simulink model "SF032A_MotTqCmdSca"  (R2013b)
settings: Solver=FixedStepDiscrete  SolverMode=SingleTasking  StartTime=0.0  StopTime=10  FixedStep=0.002  RelTol=1e-3
values from neighbouring files (symbols this model uses):
  MotTqCmdScaMax = DataDict.Calibration    [SF032A_MotTqCmdSca_DataDict.m]
  MotTqCmdScaMin = DataDict.Calibration    [SF032A_MotTqCmdSca_DataDict.m]
undefined symbols (not defined in the file or in its folder): NvmGetErrSts1
libraries: simulink x6, NxtrNvM x3, NxtrLim x2
Description:
  | The EOL Torque Command Scale function multiplies the MRFMtrTrqCmd input signal by a calibration which is set during a manufacturing
  | end of line calibration process. The calibration is provided to reduce overall system output torque variation. This scaled version of the motor
  | torque command is used by SF99B - Motor Control.
settings Model: Creator=LZDRZ1  LastModifiedBy=TZ5743
settings SolverCC: AutoInsertRateTranBlk=on  InsertRTBMode=Always
settings DataIOCC: LimitDataPoints=off  SaveFormat=Structure  ReturnWorkspaceOutputs=on
settings OptimizationCC: BlockReduction=off  InlineParams=on  ZeroExternalMemoryAtStartup=off  ZeroInternalMemoryAtStartup=off  OptimizeModelRefInitCode=on  LifeSpan=1
settings DebuggingCC: SignalInfNanChecking=error  SignalRangeChecking=warning  UnderspecifiedInitializationDetection=Simplified  SolverPrmCheckMsg=error  InheritedTsInSrcMsg=error  DiscreteInheritContinuousMsg=error  SingleTaskRateTransMsg=error  TasksWithSamePriorityMsg=error  SigSpecEnsureSampleTimeMsg=error  CheckMatrixSingularityMsg=error  ParameterUnderflowMsg=error  ParameterPrecisionLossMsg=error  ParameterTunabilityLossMsg=error  FixptConstUnderflowMsg=warning  FixptConstOverflowMsg=warning  VectorMatrixConversionMsg=error  SignalLabelMismatchMsg=error  UnconnectedInputMsg=error  UnconnectedOutputMsg=error  UnconnectedLineMsg=error  SFcnCompatibilityMsg=error  UniqueDataStoreMsg=warning  BusObjectLabelMismatch=error  RootOutportRequireBusObject=error  AssertControl=DisableAll  ModelReferenceIOMsg=error  ModelReferenceVersionMismatchMessage=warning  ModelReferenceIOMismatchMessage=error  ModelReferenceCSMismatchMessage=warning  ModelReferenceDataLoggingMessage=error  StateNameClashWarn=warning  StrictBusMsg=ErrorOnBusTreatedAsVector  NonBusSignalsTreatedAsBus=error  SFUnexpectedBacktrackingDiag=error  SFInvalidInputDataAccessInChartInitDiag=error  SFNoUnconditionalDefaultTransitionDiag=error  SFTransitionOutsideNaturalParentDiag=error  SFUnconditionalTransitionShadowingDiag=error  SFUndirectedBroadcastEventsDiag=error
settings ModelReferenceCC: ModelReferenceNumInstancesAllowed=Single
settings RTWCC: SystemTargetFile=autosar.tlc  GenCodeOnly=on  TemplateMakefile=ert_default_tmf  Description=AUTOSAR  GenerateReport=on  ProcessScript=autosar_make_rtw_hook  LaunchReport=on
settings CodeAppCC: GenerateComments=off  IgnoreCustomStorageClasses=off  CustomSymbolStrType=$N$R$M  CustomSymbolStrBlkIO=$N$M  SimulinkBlockComments=off
settings STFCustomTargetCC: ParMdlRefBuildCompliant=on  CompOptLevelCompliant=on  IncludeMdlTerminateFcn=off  CombineOutputUpdateFcns=on  SuppressErrorStatus=on  ERTFirstTimeCompliant=on  ERTCustomFileBanners=on  SupportNonFinite=off  SupportComplex=off  SupportContinuousTime=off  SupportNonInlinedSFcns=off  MATLABClassNameForMDSCustomization=Simulink.SoftwareTarget.ERTCustomization  AutosarCompliant=on  GRTInterface=off  SystemTargetFile=autosar.tlc
settings ERTTargetCC: CodeReplacementLibrary=ANSI_C  ConcurrentExecutionCompliant=off  IncludeMdlTerminateFcn=off  SuppressErrorStatus=on  SupportNonFinite=off  SupportComplex=off  ModelStepFunctionPrototypeControlCompliant=off  CPPClassGenCompliant=off  AutosarCompliant=on  InlinedParameterPlacement=NonHierarchical  ERTCustomFileTemplate=example_file_process.tlc  EnableUserReplacementTypes=on

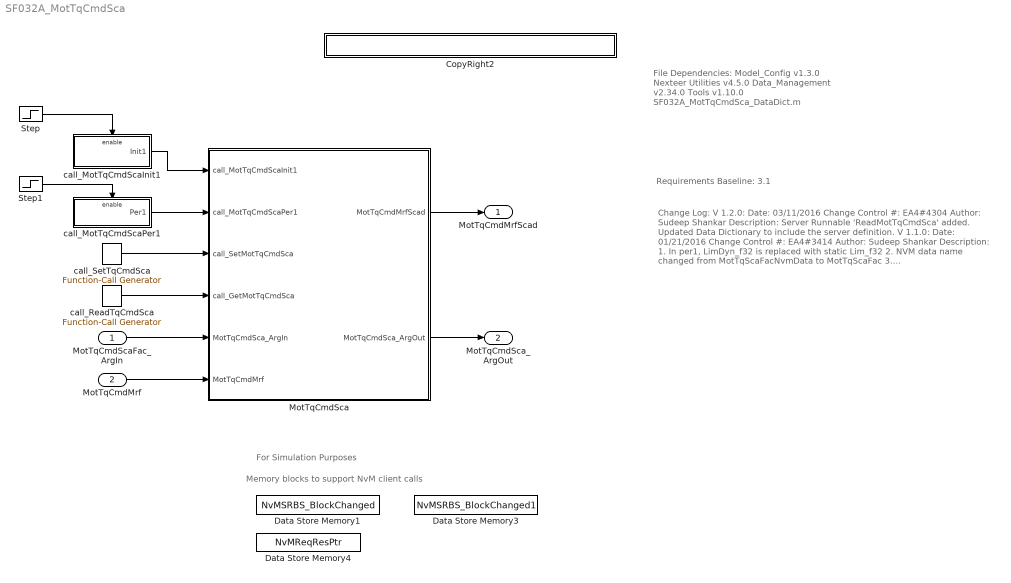
== system SF032A_MotTqCmdSca ==
  note: Change Log:
      |
      | V 1.2.0:
      | Date: 03/11/2016
      | Change Control #: EA4#4304
      | Author: Sudeep Shankar
      | Description: Server Runnable 'ReadMotTqCmdSca' added. Updated
      | Data Dictionary to include the server definition.
      |
      | V 1.1.0:
      | Date: 01/21/2016
      | Change Control #: EA4#3414
      | Author: Sudeep Shankar
      | Description:
      | 1. In per1, LimDyn_f32  is replaced with static Lim_f32
      | 2. NVM data name changed from MotTqScaFacNvmData
      |     to MotTqScaFac
      | 3. MotTqScaFacNvmData.EngInit changed from 1 to [] and ASIL
      |     level changed from 'QM' to 'D' in Data Dictionary
      | 4. SetMotTqCmdSca SrvRunnable MotTqCmdSca argument
      |     range changed in DD : EngMax = 1.1 and EngMin = 0.9
      | 5. SYSGLBPRMMOTTQCMDHILIM_MOTNWTMTR_F32
      | changed to SYSGLBPRM_MOTTQCMDHILIM_MOTNWTMTR_F32
      | 6. SYSGLBPRMMOTTQCMDLOWRLIM_MOTNWTMTR_F32
      | changed to SYSGLBPRM_MOTTQCMDLOLIM_MOTNWTMTR_F32
      |
      |
      | V 1.0.0
      | Date: 01/07/2016
      | Change Control #: EA4#2728
      | Author: Sudeep Shankar
      | Description:
      | - Initial Release Based on EA3 V 1.0.0
  note: File Dependencies:
      |
      | Model_Config v1.3.0
      | Nexteer Utilities v4.5.0
      | Data_Management v2.34.0
      | Tools v1.10.0
      | SF032A_MotTqCmdSca_DataDict.m
  note: Requirements Baseline: 3.1
  note: For Simulation Purposes
  note: Memory blocks to support NvM client calls
  MotTqCmdScaFac_ArgIn : Inport
  MotTqCmdMrf : Inport  RequirementInfo={} %GIDa_844b656b_352f_4279_ab07_8ab5443a19da  Port=2
  CopyRight2 : Subsystem  Description=|  mask(Copyright Information){none=on}
      | Copyright info block.                                               
      |                                                                     
      | Place copyright information at the top of every subsystem in design.
      mask prompts: none "No parameters"
      mask help: Place copyright information at the top of every subsystem in design.
      mask Display:
      | NxtrConf = 'Nexteer Confidential';
      | 
      | sys = bdroot; %handle for the current model ("system")
      | first = get_param(sys,'Created');
      | if(isempty(first))
      |     first = datestr(now,'yyyy');
      | else
      |     first = first(end-3:end);  %year is last four digits
      | end
      | 
      | last = get_param(sys,'LastModifiedDate');
      | if isempty(last)
      |     last = datestr(now,'yyyy');
      | else
      |     last = last(end-3:end);
      | end
      | 
      | if strcmp(first,last)
      |     fprintf('%s -- Copyright %s Nexteer',NxtrConf,first)
      | else
      |     fprintf('%s -- %s%s- %s Nexteer',NxtrConf,char(169),first,last)
      | end
  Data Store Memory1 : DataStoreMemory  DataStoreName=NvMSRBS_BlockChanged  ReadBeforeWriteMsg=warning  WriteAfterWriteMsg=warning  WriteAfterReadMsg=warning
  Data Store Memory3 : DataStoreMemory  DataStoreName=NvMSRBS_BlockChanged1  ReadBeforeWriteMsg=warning  WriteAfterWriteMsg=warning  WriteAfterReadMsg=warning
  Data Store Memory4 : DataStoreMemory  DataStoreName=NvMReqResPtr  ReadBeforeWriteMsg=warning  WriteAfterWriteMsg=warning  WriteAfterReadMsg=warning  OutDataTypeStr=double
  MotTqCmdSca : Subsystem
  Step : Step  Time=.001  Before=1  After=0  SampleTime=0
  Step1 : Step  Time=.002  SampleTime=0
  call_MotTqCmdScaInit1 : Subsystem  TreatAsAtomicUnit=on
  call_MotTqCmdScaPer1 : Subsystem  TreatAsAtomicUnit=on
  call_ReadTqCmdSca : simulink/Ports & Subsystems/Function-Call Generator  sample_time=.004  numberOfIterations=1
  call_SetTqCmdSca : simulink/Ports & Subsystems/Function-Call Generator  sample_time=.004  numberOfIterations=1
  MotTqCmdMrfScad : Outport
  MotTqCmdSca_ArgOut : Outport  Port=2
  wires:
  MotTqCmdMrf/1 -> MotTqCmdSca/6(MotTqCmdMrf)
  Step/1 -> call_MotTqCmdScaInit1/Enable
  call_MotTqCmdScaInit1/1(Init1) -> MotTqCmdSca/1(call_MotTqCmdScaInit1)
  call_MotTqCmdScaPer1/1(Per1) -> MotTqCmdSca/2(call_MotTqCmdScaPer1)
  Step1/1 -> call_MotTqCmdScaPer1/Enable
  call_SetTqCmdSca/1 -> MotTqCmdSca/3(call_SetMotTqCmdSca)
  MotTqCmdSca/1(MotTqCmdMrfScad) -> MotTqCmdMrfScad/1
  MotTqCmdScaFac_ArgIn/1 -> MotTqCmdSca/5(MotTqCmdSca_ArgIn)
  call_ReadTqCmdSca/1 -> MotTqCmdSca/4(call_GetMotTqCmdSca)
  MotTqCmdSca/2(MotTqCmdSca_ArgOut) -> MotTqCmdSca_ArgOut/1

== system SF032A_MotTqCmdSca/CopyRight2 ==

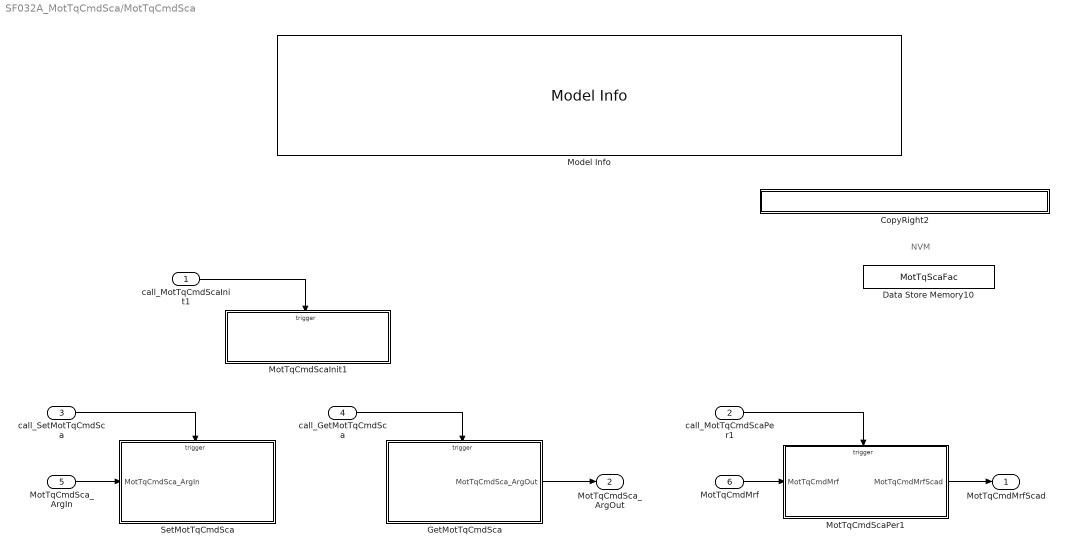
== system SF032A_MotTqCmdSca/MotTqCmdSca ==
  note: NVM
  call_MotTqCmdScaInit1 : Inport
  call_MotTqCmdScaPer1 : Inport  Port=2
  call_SetMotTqCmdSca : Inport  RequirementInfo={} %GIDa_c34c7997_18b4_40d6_8eff_4a1c6cbbe59c  Port=3
  call_GetMotTqCmdSca : Inport  RequirementInfo={} %GIDa_22899b86_5e5a_4bad_994d_b3055ed379bb  Port=4
  MotTqCmdSca_ArgIn : Inport  RequirementInfo="{'linktype_rmi_doors' '0000a539 (/E-STEER Core/SubSystem Specifications/Application Functions/SF032A EOL Torque Command Scale)' '#SF032A_40' 'true' 'REQ:  SF032A_40' '' } %GIDa_79343901_a042_40db_a967_ce644dcbc3fd"  Port=5
  MotTqCmdMrf : Inport  RequirementInfo="{'linktype_rmi_doors' '0000a539 (/E-STEER Core/SubSystem Specifications/Application Functions/SF032A EOL Torque Command Scale)' '#SF032A_9' 'true' 'REQ:  SF032A_9' '' } %GIDa_c4547729_827d_4a2a_8a7c_5db9c8d83c52"  Port=6
  CopyRight2 : Subsystem  Description=|  mask(Copyright Information){none=on}
      | Copyright info block.                                               
      |                                                                     
      | Place copyright information at the top of every subsystem in design.
      mask prompts: none "No parameters"
      mask help: Place copyright information at the top of every subsystem in design.
      mask Display:
      | NxtrConf = 'Nexteer Confidential';
      | 
      | sys = bdroot; %handle for the current model ("system")
      | first = get_param(sys,'Created');
      | if(isempty(first))
      |     first = datestr(now,'yyyy');
      | else
      |     first = first(end-3:end);  %year is last four digits
      | end
      | 
      | last = get_param(sys,'LastModifiedDate');
      | if isempty(last)
      |     last = datestr(now,'yyyy');
      | else
      |     last = last(end-3:end);
      | end
      | 
      | if strcmp(first,last)
      |     fprintf('%s -- Copyright %s Nexteer',NxtrConf,first)
      | else
      |     fprintf('%s -- %s%s- %s Nexteer',NxtrConf,char(169),first,last)
      | end
  Data Store Memory10 : DataStoreMemory  DataStoreName=MotTqScaFac  InitialValue=[]  StateMustResolveToSignalObject=on
  GetMotTqCmdSca : Subsystem
  Model Info : simulink/Model-Wide Utilities/Model Info  InitialBlockCM=None  Frame=on  DisplayStringWithTags=|  HorizontalTextAlignment=Left  LeftAlignmentValue=0.02  SourceBlockDiagram=SF032A_MotTqCmdSca  TagMaxNumber=20
      | SF032A - Torque Command Scale
      | Version 1.2.0
      | 
      | Created by Siddharth Ballal on %<Created>.
      | Last Modified on %<LastModificationDate>.
      | 
      | Description:
      | %<Description>
  MotTqCmdScaInit1 : Subsystem
  MotTqCmdScaPer1 : Subsystem
  SetMotTqCmdSca : Subsystem
  MotTqCmdMrfScad : Outport  RequirementInfo="{'linktype_rmi_doors' '0000a539 (/E-STEER Core/SubSystem Specifications/Application Functions/SF032A EOL Torque Command Scale)' '#SF032A_11' 'true' 'REQ:  SF032A_11' '' } %GIDa_399fda8a_bea6_4221_a883_de3914a08159"
  MotTqCmdSca_ArgOut : Outport  RequirementInfo="{'linktype_rmi_doors' '0000a539 (/E-STEER Core/SubSystem Specifications/Application Functions/SF032A EOL Torque Command Scale)' '#SF032A_11' 'true' 'REQ:  SF032A_11' '' ; 'linktype_rmi_doors' '0000a539 (/E-STEER Core/SubSystem Specifications/Application Functions/SF032A EOL Torque Command Scale)' '#SF032A_30' 'true' 'REQ:  SF032A_30' '' } %GIDa_1b173d9c_2484_4f48_ad4f_c1a7996ff12f"  Port=2
  wires:
  call_MotTqCmdScaPer1/1 -> MotTqCmdScaPer1/Trigger
  MotTqCmdScaPer1/1(MotTqCmdMrfScad) -> MotTqCmdMrfScad/1
  call_MotTqCmdScaInit1/1 -> MotTqCmdScaInit1/Trigger
  MotTqCmdMrf/1 -> MotTqCmdScaPer1/1(MotTqCmdMrf)
  call_SetMotTqCmdSca/1 -> SetMotTqCmdSca/Trigger
  MotTqCmdSca_ArgIn/1 -> SetMotTqCmdSca/1(MotTqCmdSca_ArgIn)
  call_GetMotTqCmdSca/1 -> GetMotTqCmdSca/Trigger
  GetMotTqCmdSca/1(MotTqCmdSca_ArgOut) -> MotTqCmdSca_ArgOut/1

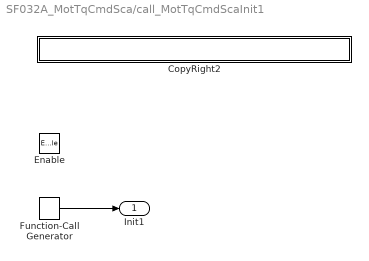
== system SF032A_MotTqCmdSca/call_MotTqCmdScaInit1 ==
  Enable : EnablePort
  CopyRight2 : Subsystem  Description=|  mask(Copyright Information){none=on}
      | Copyright info block.                                               
      |                                                                     
      | Place copyright information at the top of every subsystem in design.
      mask prompts: none "No parameters"
      mask help: Place copyright information at the top of every subsystem in design.
      mask Display:
      | NxtrConf = 'Nexteer Confidential';
      | 
      | sys = bdroot; %handle for the current model ("system")
      | first = get_param(sys,'Created');
      | if(isempty(first))
      |     first = datestr(now,'yyyy');
      | else
      |     first = first(end-3:end);  %year is last four digits
      | end
      | 
      | last = get_param(sys,'LastModifiedDate');
      | if isempty(last)
      |     last = datestr(now,'yyyy');
      | else
      |     last = last(end-3:end);
      | end
      | 
      | if strcmp(first,last)
      |     fprintf('%s -- Copyright %s Nexteer',NxtrConf,first)
      | else
      |     fprintf('%s -- %s%s- %s Nexteer',NxtrConf,char(169),first,last)
      | end
  Function-Call Generator : simulink/Ports & Subsystems/Function-Call Generator  sample_time=.004  numberOfIterations=1
  Init1 : Outport
  wires:
  Function-Call Generator/1 -> Init1/1

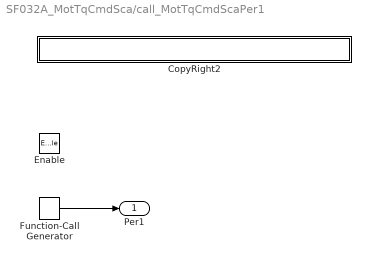
== system SF032A_MotTqCmdSca/call_MotTqCmdScaPer1 ==
  Enable : EnablePort
  CopyRight2 : Subsystem  Description=|  mask(Copyright Information){none=on}
      | Copyright info block.                                               
      |                                                                     
      | Place copyright information at the top of every subsystem in design.
      mask prompts: none "No parameters"
      mask help: Place copyright information at the top of every subsystem in design.
      mask Display:
      | NxtrConf = 'Nexteer Confidential';
      | 
      | sys = bdroot; %handle for the current model ("system")
      | first = get_param(sys,'Created');
      | if(isempty(first))
      |     first = datestr(now,'yyyy');
      | else
      |     first = first(end-3:end);  %year is last four digits
      | end
      | 
      | last = get_param(sys,'LastModifiedDate');
      | if isempty(last)
      |     last = datestr(now,'yyyy');
      | else
      |     last = last(end-3:end);
      | end
      | 
      | if strcmp(first,last)
      |     fprintf('%s -- Copyright %s Nexteer',NxtrConf,first)
      | else
      |     fprintf('%s -- %s%s- %s Nexteer',NxtrConf,char(169),first,last)
      | end
  Function-Call Generator : simulink/Ports & Subsystems/Function-Call Generator  sample_time=.004  numberOfIterations=1
  Per1 : Outport
  wires:
  Function-Call Generator/1 -> Per1/1

== system SF032A_MotTqCmdSca/MotTqCmdSca/CopyRight2 ==

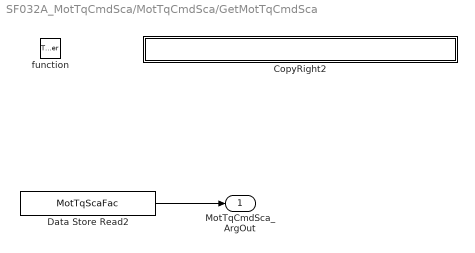
== system SF032A_MotTqCmdSca/MotTqCmdSca/GetMotTqCmdSca ==
  function : TriggerPort  TriggerType=function-call
  CopyRight2 : Subsystem  Description=|  mask(Copyright Information){none=on}
      | Copyright info block.                                               
      |                                                                     
      | Place copyright information at the top of every subsystem in design.
      mask prompts: none "No parameters"
      mask help: Place copyright information at the top of every subsystem in design.
      mask Display:
      | NxtrConf = 'Nexteer Confidential';
      | 
      | sys = bdroot; %handle for the current model ("system")
      | first = get_param(sys,'Created');
      | if(isempty(first))
      |     first = datestr(now,'yyyy');
      | else
      |     first = first(end-3:end);  %year is last four digits
      | end
      | 
      | last = get_param(sys,'LastModifiedDate');
      | if isempty(last)
      |     last = datestr(now,'yyyy');
      | else
      |     last = last(end-3:end);
      | end
      | 
      | if strcmp(first,last)
      |     fprintf('%s -- Copyright %s Nexteer',NxtrConf,first)
      | else
      |     fprintf('%s -- %s%s- %s Nexteer',NxtrConf,char(169),first,last)
      | end
  Data Store Read2 : DataStoreRead  RequirementInfo="{'linktype_rmi_doors' '0000a539 (/E-STEER Core/SubSystem Specifications/Application Functions/SF032A EOL Torque Command Scale)' '#SF032A_50' 'true' 'REQ:  SF032A_50' '' ; 'linktype_rmi_doors' '0000a539 (/E-STEER Core/SubSystem Specifications/Application Functions/SF032A EOL Torque Command Scale)' '#SF032A_51' 'true' 'REQ:  SF032A_51' '' } %GIDa_04a98167_9d79_4de8_93b5_a58e6ecf13fd"  DataStoreName=MotTqScaFac
  MotTqCmdSca_ArgOut : Outport  RequirementInfo="{'linktype_rmi_doors' '0000a539 (/E-STEER Core/SubSystem Specifications/Application Functions/SF032A EOL Torque Command Scale)' '#SF032A_50' 'true' 'REQ:  SF032A_50' '' } %GIDa_56e9da4a_e100_4f0b_b52f_b1954dfd6c3d"
  wires:
  Data Store Read2/1 -> MotTqCmdSca_ArgOut/1

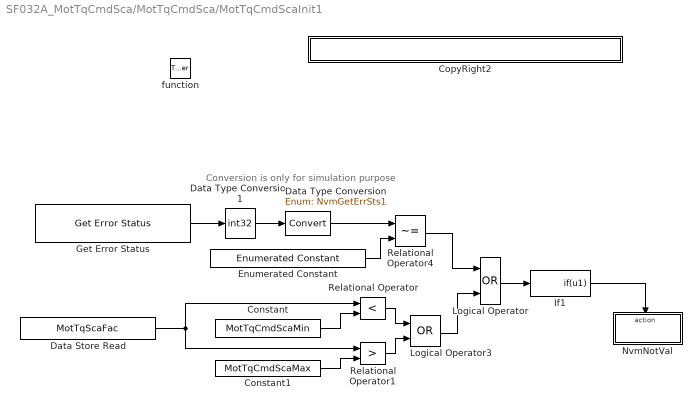
== system SF032A_MotTqCmdSca/MotTqCmdSca/MotTqCmdScaInit1 ==
  note: Conversion is only for simulation purpose
  function : TriggerPort  TriggerType=function-call
  Constant : Constant  RequirementInfo="{'linktype_rmi_doors' '0000a539 (/E-STEER Core/SubSystem Specifications/Application Functions/SF032A EOL Torque Command Scale)' '#SF032A_48' 'true' 'REQ:  SF032A_48' '' } %GIDa_02276521_3c3d_4cdd_8a72_3fdbb82cd493"  Value=MotTqCmdScaMin
  Constant1 : Constant  RequirementInfo="{'linktype_rmi_doors' '0000a539 (/E-STEER Core/SubSystem Specifications/Application Functions/SF032A EOL Torque Command Scale)' '#SF032A_48' 'true' 'REQ:  SF032A_48' '' } %GIDa_09147d74_3ee4_4904_9485_0fa6e15eda40"  Value=MotTqCmdScaMax
  CopyRight2 : Subsystem  Description=|  mask(Copyright Information){none=on}
      | Copyright info block.                                               
      |                                                                     
      | Place copyright information at the top of every subsystem in design.
      mask prompts: none "No parameters"
      mask help: Place copyright information at the top of every subsystem in design.
      mask Display:
      | NxtrConf = 'Nexteer Confidential';
      | 
      | sys = bdroot; %handle for the current model ("system")
      | first = get_param(sys,'Created');
      | if(isempty(first))
      |     first = datestr(now,'yyyy');
      | else
      |     first = first(end-3:end);  %year is last four digits
      | end
      | 
      | last = get_param(sys,'LastModifiedDate');
      | if isempty(last)
      |     last = datestr(now,'yyyy');
      | else
      |     last = last(end-3:end);
      | end
      | 
      | if strcmp(first,last)
      |     fprintf('%s -- Copyright %s Nexteer',NxtrConf,first)
      | else
      |     fprintf('%s -- %s%s- %s Nexteer',NxtrConf,char(169),first,last)
      | end
  Data Store Read : DataStoreRead  RequirementInfo="{'linktype_rmi_doors' '0000a539 (/E-STEER Core/SubSystem Specifications/Application Functions/SF032A EOL Torque Command Scale)' '#SF032A_48' 'true' 'REQ:  SF032A_48' '' } %GIDa_eb96d928_3db0_4476_aaab_f2b08e018012"  DataStoreName=MotTqScaFac
  Data Type Conversion : DataTypeConversion  RequirementInfo="{'linktype_rmi_doors' '0000a539 (/E-STEER Core/SubSystem Specifications/Application Functions/SF032A EOL Torque Command Scale)' '#SF032A_47' 'true' 'REQ:  SF032A_47' '' } %GIDa_7da365b6_545f_4e3b_8f8e_b7fa76fed2e1"  OutDataTypeStr=Enum: NvmGetErrSts1
  Data Type Conversion1 : DataTypeConversion  RequirementInfo="{'linktype_rmi_doors' '0000a539 (/E-STEER Core/SubSystem Specifications/Application Functions/SF032A EOL Torque Command Scale)' '#SF032A_47' 'true' 'REQ:  SF032A_47' '' } %GIDa_218a8008_1fb3_4f0f_b469_2e11fb8f2ba7"  OutDataTypeStr=int32
  Enumerated Constant : simulink/Sources/Enumerated Constant  RequirementInfo="{'linktype_rmi_doors' '0000a539 (/E-STEER Core/SubSystem Specifications/Application Functions/SF032A EOL Torque Command Scale)' '#SF032A_47' 'true' 'REQ:  SF032A_47' '' } %GIDa_47049bff_eea1_4ad9_9652_1bea39283af9"  OutDataTypeStr=Enum: NvmGetErrSts1  Value=NvmGetErrSts1.REQUEST_OK  SampleTime=inf
  Get Error Status : NxtrNvM/Get Error Status  RequirementInfo="{'linktype_rmi_doors' '0000a539 (/E-STEER Core/SubSystem Specifications/Application Functions/SF032A EOL Torque Command Scale)' '#SF032A_47' 'true' 'REQ:  SF032A_47' '' } %GIDa_ac713a46_7264_462b_9524_2b7bcd81a9ca"  FuncName=Get Error Status  NvMBlockName=MotTqScaFac  VoidFuncRtn=on  ReqResPtr_DSN=NvMReqResPtr  Return_DSN=NvMGES_ReqResPtr
      settings: AttributesFormatString=%<FuncName>
  If1 : If  RequirementInfo={} %GIDa_9ad9b513_6643_45ca_bd66_0d9ba3219669  Priority=0  IfExpression=u1  ShowElse=off
  Logical Operator : Logic  RequirementInfo="{'linktype_rmi_doors' '0000a539 (/E-STEER Core/SubSystem Specifications/Application Functions/SF032A EOL Torque Command Scale)' '#SF032A_48' 'true' 'REQ:  SF032A_48' '' ; 'linktype_rmi_doors' '0000a539 (/E-STEER Core/SubSystem Specifications/Application Functions/SF032A EOL Torque Command Scale)' '#SF032A_47' 'true' 'REQ:  SF032A_47' '' } %GIDa_74286b1a_fff6_470a_a7a8_1c80ceb0305d"  Operator=OR  AllPortsSameDT=off  OutDataTypeStr=boolean
  Logical Operator3 : Logic  RequirementInfo="{'linktype_rmi_doors' '0000a539 (/E-STEER Core/SubSystem Specifications/Application Functions/SF032A EOL Torque Command Scale)' '#SF032A_48' 'true' 'REQ:  SF032A_48' '' } %GIDa_1918f32a_8081_4063_b730_06fad75d4206"  Operator=OR  AllPortsSameDT=off  OutDataTypeStr=boolean
  NvmNotVal : Subsystem  RequirementInfo="{'linktype_rmi_doors' '0000a539 (/E-STEER Core/SubSystem Specifications/Application Functions/SF032A EOL Torque Command Scale)' '#SF032A_47' 'true' 'REQ:  SF032A_47' '' ; 'linktype_rmi_doors' '0000a539 (/E-STEER Core/SubSystem Specifications/Application Functions/SF032A EOL Torque Command Scale)' '#SF032A_48' 'true' 'REQ:  SF032A_48' '' } %GIDa_95ece82d_80c3_4582_9fd5_5f3c695684e4"  TreatAsAtomicUnit=on
  Relational Operator : RelationalOperator  RequirementInfo="{'linktype_rmi_doors' '0000a539 (/E-STEER Core/SubSystem Specifications/Application Functions/SF032A EOL Torque Command Scale)' '#SF032A_48' 'true' 'REQ:  SF032A_48' '' } %GIDa_4574bc11_8b95_4c9a_9b5e_35c5069dd5b0"  Operator=<  OutDataTypeStr=boolean
  Relational Operator1 : RelationalOperator  RequirementInfo="{'linktype_rmi_doors' '0000a539 (/E-STEER Core/SubSystem Specifications/Application Functions/SF032A EOL Torque Command Scale)' '#SF032A_48' 'true' 'REQ:  SF032A_48' '' } %GIDa_c74274c9_a218_4ff9_b7e5_7d169d276d93"  Operator=>  OutDataTypeStr=boolean
  Relational Operator4 : RelationalOperator  RequirementInfo="{'linktype_rmi_doors' '0000a539 (/E-STEER Core/SubSystem Specifications/Application Functions/SF032A EOL Torque Command Scale)' '#SF032A_47' 'true' 'REQ:  SF032A_47' '' } %GIDa_140cc552_aeaa_4d20_9169_4962e472b60d"  Operator=~=  OutDataTypeStr=boolean
  wires:
  If1/1 -> NvmNotVal/Action
  Relational Operator4/1 -> Logical Operator/1
  Enumerated Constant/1 -> Relational Operator4/2
  Data Type Conversion/1 -> Relational Operator4/1
  Get Error Status/1 -> Data Type Conversion1/1
  Data Type Conversion1/1 -> Data Type Conversion/1
  Logical Operator/1 -> If1/1
  Constant/1 -> Relational Operator/2
  Constant1/1 -> Relational Operator1/2
  Relational Operator/1 -> Logical Operator3/1
  Relational Operator1/1 -> Logical Operator3/2
  Data Store Read/1 -> Relational Operator1/1, Relational Operator/1
  Logical Operator3/1 -> Logical Operator/2

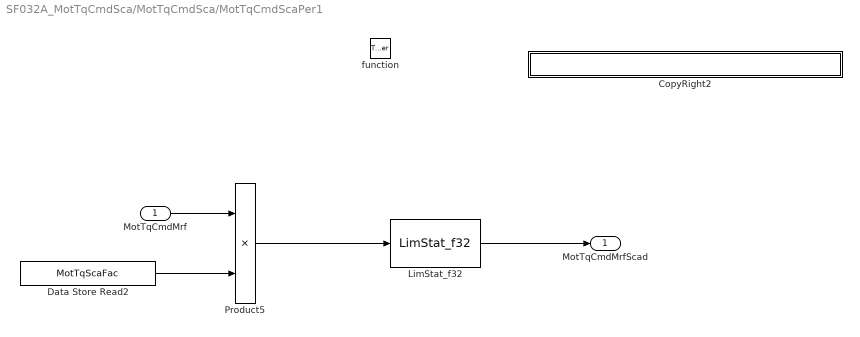
== system SF032A_MotTqCmdSca/MotTqCmdSca/MotTqCmdScaPer1 ==
  MotTqCmdMrf : Inport  RequirementInfo="{'linktype_rmi_doors' '0000a539 (/E-STEER Core/SubSystem Specifications/Application Functions/SF032A EOL Torque Command Scale)' '#SF032A_34' 'true' 'REQ:  SF032A_34' '' } %GIDa_0583ffa4_69ee_4da4_a225_24c428f6b940"
  function : TriggerPort  TriggerType=function-call
  CopyRight2 : Subsystem  Description=|  mask(Copyright Information){none=on}
      | Copyright info block.                                               
      |                                                                     
      | Place copyright information at the top of every subsystem in design.
      mask prompts: none "No parameters"
      mask help: Place copyright information at the top of every subsystem in design.
      mask Display:
      | NxtrConf = 'Nexteer Confidential';
      | 
      | sys = bdroot; %handle for the current model ("system")
      | first = get_param(sys,'Created');
      | if(isempty(first))
      |     first = datestr(now,'yyyy');
      | else
      |     first = first(end-3:end);  %year is last four digits
      | end
      | 
      | last = get_param(sys,'LastModifiedDate');
      | if isempty(last)
      |     last = datestr(now,'yyyy');
      | else
      |     last = last(end-3:end);
      | end
      | 
      | if strcmp(first,last)
      |     fprintf('%s -- Copyright %s Nexteer',NxtrConf,first)
      | else
      |     fprintf('%s -- %s%s- %s Nexteer',NxtrConf,char(169),first,last)
      | end
  Data Store Read2 : DataStoreRead  RequirementInfo="{'linktype_rmi_doors' '0000a539 (/E-STEER Core/SubSystem Specifications/Application Functions/SF032A EOL Torque Command Scale)' '#SF032A_34' 'true' 'REQ:  SF032A_34' '' } %GIDa_19ef9106_7afa_4327_be19_f515e5f3f95e"  DataStoreName=MotTqScaFac
  LimStat_f32 : NxtrLim/LimStat_f32  RequirementInfo="{'linktype_rmi_doors' '0000a539 (/E-STEER Core/SubSystem Specifications/Application Functions/SF032A EOL Torque Command Scale)' '#SF032A_36' 'true' 'REQ:  SF032A_36' '' } %GIDa_38d851c1_1888_41cd_a2aa_fef940cb6c88"  LoLim=SYSGLBPRM_MOTTQCMDLOLIM_MOTNWTMTR_F32  HiLim=SYSGLBPRM_MOTTQCMDHILIM_MOTNWTMTR_F32
      settings: AttributesFormatString=|
      | Low Limit: %<LoLim>
      | High Limit:%<HiLim>
  Product5 : Product  RequirementInfo="{'linktype_rmi_doors' '0000a539 (/E-STEER Core/SubSystem Specifications/Application Functions/SF032A EOL Torque Command Scale)' '#SF032A_34' 'true' 'REQ:  SF032A_34' '' } %GIDa_3a44c5c6_bfdd_409e_b6a6_14570aaf2a05"  RndMeth=Zero
  MotTqCmdMrfScad : Outport  RequirementInfo={} %GIDa_d12e8a64_7da5_445a_bb0d_8047151ae747
  wires:
  Product5/1 -> LimStat_f32/1
  MotTqCmdMrf/1 -> Product5/1
  LimStat_f32/1 -> MotTqCmdMrfScad/1
  Data Store Read2/1 -> Product5/2

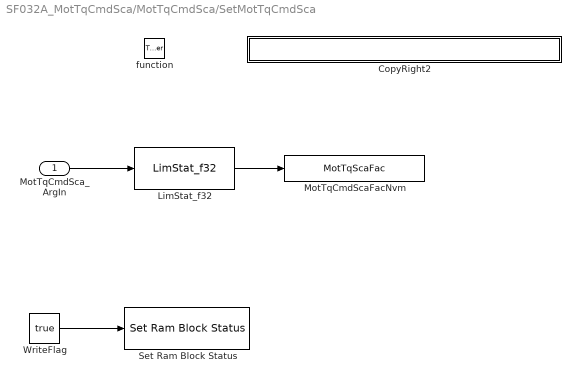
== system SF032A_MotTqCmdSca/MotTqCmdSca/SetMotTqCmdSca ==
  MotTqCmdSca_ArgIn : Inport  RequirementInfo={} %GIDa_e805bfa1_5bb2_43ee_8e7a_3ba8b8a60b42
  function : TriggerPort  TriggerType=function-call
  CopyRight2 : Subsystem  Description=|  mask(Copyright Information){none=on}
      | Copyright info block.                                               
      |                                                                     
      | Place copyright information at the top of every subsystem in design.
      mask prompts: none "No parameters"
      mask help: Place copyright information at the top of every subsystem in design.
      mask Display:
      | NxtrConf = 'Nexteer Confidential';
      | 
      | sys = bdroot; %handle for the current model ("system")
      | first = get_param(sys,'Created');
      | if(isempty(first))
      |     first = datestr(now,'yyyy');
      | else
      |     first = first(end-3:end);  %year is last four digits
      | end
      | 
      | last = get_param(sys,'LastModifiedDate');
      | if isempty(last)
      |     last = datestr(now,'yyyy');
      | else
      |     last = last(end-3:end);
      | end
      | 
      | if strcmp(first,last)
      |     fprintf('%s -- Copyright %s Nexteer',NxtrConf,first)
      | else
      |     fprintf('%s -- %s%s- %s Nexteer',NxtrConf,char(169),first,last)
      | end
  LimStat_f32 : NxtrLim/LimStat_f32  RequirementInfo="{'linktype_rmi_doors' '0000a539 (/E-STEER Core/SubSystem Specifications/Application Functions/SF032A EOL Torque Command Scale)' '#SF032A_13' 'true' 'REQ:  SF032A_13' '' ; 'linktype_rmi_doors' '0000a539 (/E-STEER Core/SubSystem Specifications/Application Functions/SF032A EOL Torque Command Scale)' '#SF032A_14' 'true' 'REQ:  SF032A_14' '' ; 'linktype_rmi_doors' '0000a539 (/E-STEER Core/SubSystem Specifications/Application Functions/SF032A EOL Torque Command Scale)' '#SF032A_45' 'true' 'REQ:  SF032A_45' '' } %GIDa_4d405e5b_1b19_4d3f_8e83_00be4e20b553"  LoLim=MotTqCmdScaMin  HiLim=MotTqCmdScaMax
      settings: AttributesFormatString=|
      | Low Limit: %<LoLim>
      | High Limit:%<HiLim>
  MotTqCmdScaFacNvm : DataStoreWrite  RequirementInfo={} %GIDa_19d58e6c_0ebc_49d7_9780_924a421f6d31  DataStoreName=MotTqScaFac
  Set Ram Block Status : NxtrNvM/Set Ram Block Status  RequirementInfo={} %GIDa_02651dc8_91ce_4129_b8d9_36b9fab867e3  FuncName=Set Ram Block Status  NvMBlockName=MotTqScaFac  VoidFuncRtn=on  BlockChanged_DSN=NvMSRBS_BlockChanged1  Return_DSN=NvMSRBS_Return1
      settings: AttributesFormatString=%<FuncName>
  WriteFlag : Constant  RequirementInfo={} %GIDa_0417db9b_1287_463d_8a9a_034ae56dd04c  Value=true  OutDataTypeStr=boolean
      settings: AttributesFormatString=%<OutDataTypeStr>
  wires:
  MotTqCmdSca_ArgIn/1 -> LimStat_f32/1
  WriteFlag/1 -> Set Ram Block Status/1
  LimStat_f32/1 -> MotTqCmdScaFacNvm/1

== system SF032A_MotTqCmdSca/call_MotTqCmdScaInit1/CopyRight2 ==

== system SF032A_MotTqCmdSca/call_MotTqCmdScaPer1/CopyRight2 ==

== system SF032A_MotTqCmdSca/MotTqCmdSca/GetMotTqCmdSca/CopyRight2 ==

== system SF032A_MotTqCmdSca/MotTqCmdSca/MotTqCmdScaInit1/CopyRight2 ==

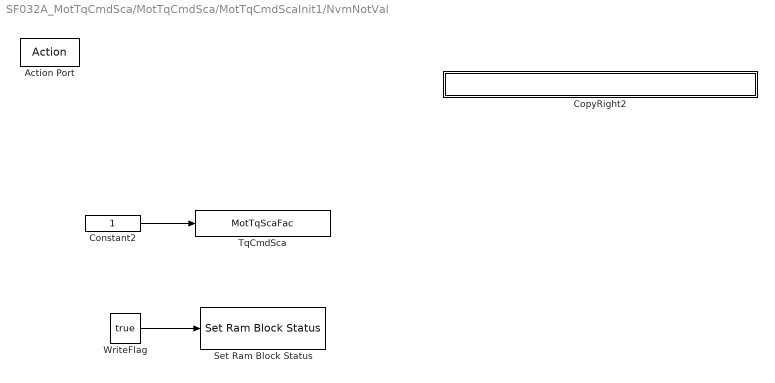
== system SF032A_MotTqCmdSca/MotTqCmdSca/MotTqCmdScaInit1/NvmNotVal ==
  Action Port : ActionPort  ActionType=then
  Constant2 : Constant  RequirementInfo={} %GIDa_8675f7c9_68cb_432e_94f8_a35779b41f30  OutDataTypeStr=single
      settings: AttributesFormatString=%<OutDataTypeStr>
  CopyRight2 : Subsystem  Description=|  mask(Copyright Information){none=on}
      | Copyright info block.                                               
      |                                                                     
      | Place copyright information at the top of every subsystem in design.
      mask prompts: none "No parameters"
      mask help: Place copyright information at the top of every subsystem in design.
      mask Display:
      | NxtrConf = 'Nexteer Confidential';
      | 
      | sys = bdroot; %handle for the current model ("system")
      | first = get_param(sys,'Created');
      | if(isempty(first))
      |     first = datestr(now,'yyyy');
      | else
      |     first = first(end-3:end);  %year is last four digits
      | end
      | 
      | last = get_param(sys,'LastModifiedDate');
      | if isempty(last)
      |     last = datestr(now,'yyyy');
      | else
      |     last = last(end-3:end);
      | end
      | 
      | if strcmp(first,last)
      |     fprintf('%s -- Copyright %s Nexteer',NxtrConf,first)
      | else
      |     fprintf('%s -- %s%s- %s Nexteer',NxtrConf,char(169),first,last)
      | end
  Set Ram Block Status : NxtrNvM/Set Ram Block Status  RequirementInfo={} %GIDa_ad5f78b3_411f_4d65_9eb7_8c3337ca78f1  FuncName=Set Ram Block Status  NvMBlockName=MotTqScaFac  VoidFuncRtn=on  BlockChanged_DSN=NvMSRBS_BlockChanged  Return_DSN=NvMSRBS_Return
      settings: AttributesFormatString=%<FuncName>
  TqCmdSca : DataStoreWrite  RequirementInfo={} %GIDa_06d8551b_8593_468a_805a_1a5cba3dcbe6  DataStoreName=MotTqScaFac
  WriteFlag : Constant  RequirementInfo={} %GIDa_b3368da2_c73f_4f9d_b8fc_67e8bbf63e57  Value=true  OutDataTypeStr=boolean
      settings: AttributesFormatString=%<OutDataTypeStr>
  wires:
  Constant2/1 -> TqCmdSca/1
  WriteFlag/1 -> Set Ram Block Status/1

== system SF032A_MotTqCmdSca/MotTqCmdSca/MotTqCmdScaPer1/CopyRight2 ==

== system SF032A_MotTqCmdSca/MotTqCmdSca/SetMotTqCmdSca/CopyRight2 ==

== system SF032A_MotTqCmdSca/MotTqCmdSca/MotTqCmdScaInit1/NvmNotVal/CopyRight2 ==
